simulink model "BeamSimulink_Question2_58282386"  (R2024b)
settings: Solver=VariableStepAuto  StartTime=0.0  StopTime=10.0  RelTol=1e-3
libraries: simulink x1
settings Model: Creator=nmfuma  LastModifiedBy=nmfuma

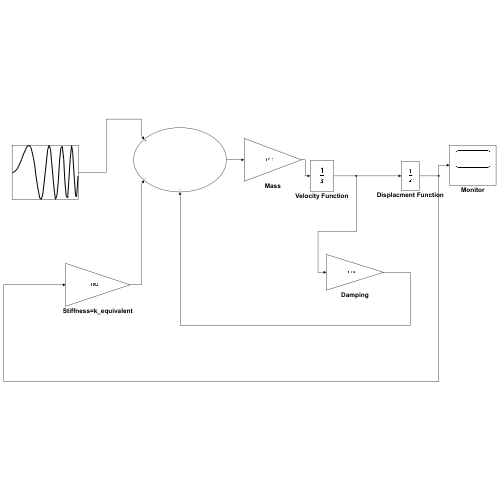
[thumbnail: Simulink's stored preview of the top-level diagram]
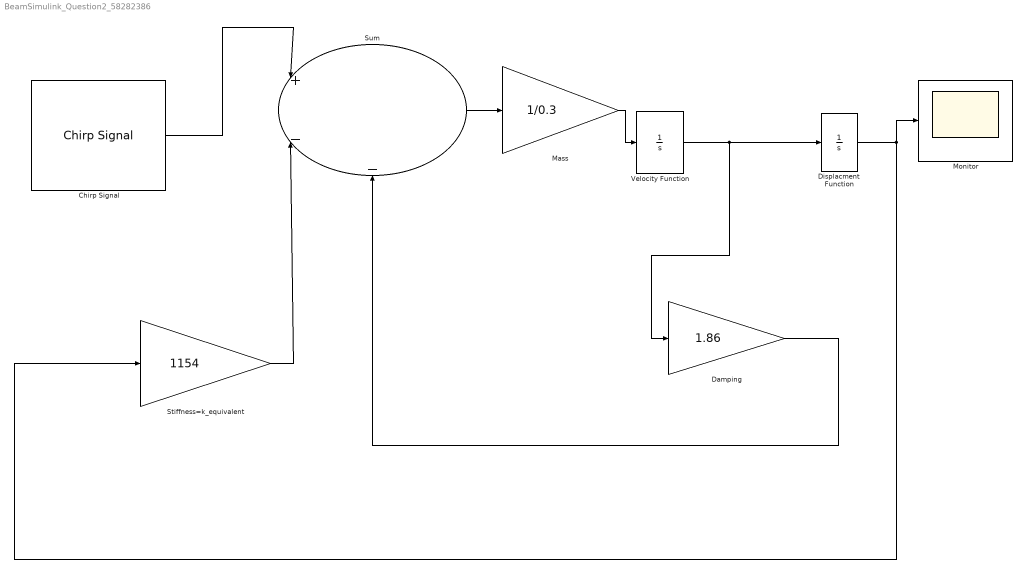
== system BeamSimulink_Question2_58282386 ==
  Chirp Signal : simulink/Sources/Chirp Signal  f1=0  T=10  f2=10
  Damping : Gain  Gain=1.86
  Displacment Function : Integrator
  Mass : Gain  Gain=1/0.3
  Monitor : Scope
  Stiffness=k_equivalent : Gain  Gain=1154
  Sum : Sum  Inputs=|+--
  Velocity Function : Integrator
  wires:
  Mass/1 -> Velocity Function/1
  Chirp Signal/1 -> Sum/1
  Sum/1 -> Mass/1
  Displacment Function/1 -> Monitor/1, Stiffness=k_equivalent/1
  Velocity Function/1 -> Displacment Function/1, Damping/1
  Stiffness=k_equivalent/1 -> Sum/2
  Damping/1 -> Sum/3
